simulink model "controller_2014B"  (R2014b)
settings: Solver=ode45  StartTime=0.0  StopTime=sim_run  FixedStep=0.001  RelTol=1e-3
InitFcn:
  | zh = 0.01;
undefined symbols (not defined in the file): Standard_Devices, UDP_Protocol, zh_step
libraries: rtwinlib x6, simulink x4, dspnetwork x2
settings Model: Creator=Lenka  LastModifiedBy=petrhomolka
settings DebuggingCC: FrameProcessingCompatibilityMsg=error

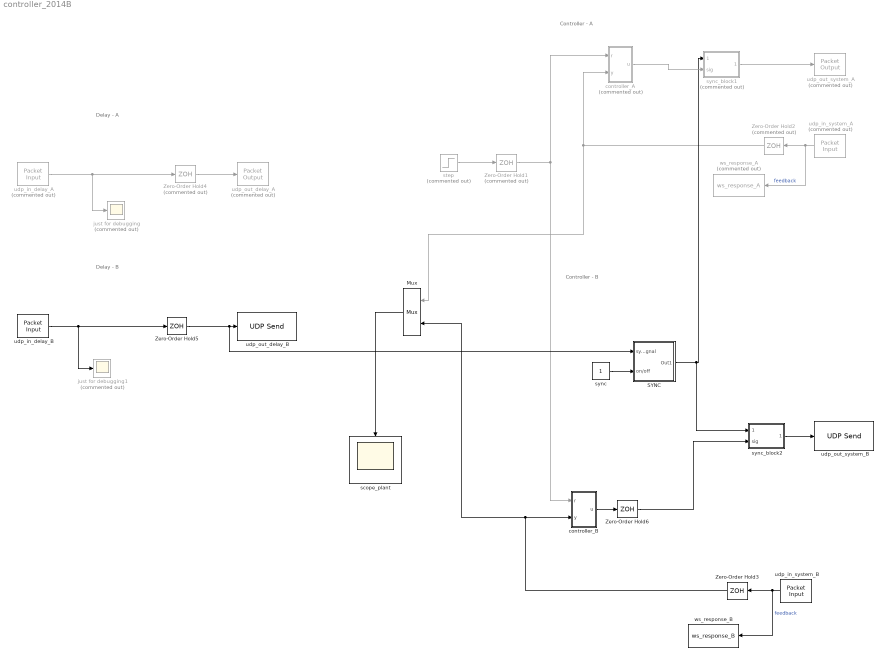
== system controller_2014B ==
  note: Controller - B
  note: Controller - A
  note: Delay - A
  note: Delay - B
  Mux : Mux  Inputs=2
  SYNC : Subsystem
  Zero-Order Hold1 : ZeroOrderHold  Commented=on  SampleTime=zh_step
  Zero-Order Hold2 : ZeroOrderHold  Commented=on  SampleTime=zh_step
  Zero-Order Hold3 : ZeroOrderHold  SampleTime=zh_step
  Zero-Order Hold4 : ZeroOrderHold  Commented=on  SampleTime=zh_step
  Zero-Order Hold5 : ZeroOrderHold  SampleTime=zh_step
  Zero-Order Hold6 : ZeroOrderHold  SampleTime=zh_step
  controller_A : Subsystem  Commented=on
  controller_B : Subsystem
  just for debugging : Scope  Commented=on
      settings: TimeRange=auto  LimitDataPoints=on  MaxDataPoints=5000  SaveToWorkspace=off  YMin=-10  YMax=10  SampleTime=-1  DataFormat=Array
  just for debugging1 : Scope  Commented=on
      settings: TimeRange=auto  LimitDataPoints=on  MaxDataPoints=5000  SaveToWorkspace=off  SaveName=ScopeData2  YMin=-10  YMax=10  SampleTime=-1  DataFormat=Array
  scope_plant : Scope
      settings: TimeRange=auto  ShowLegends=on  MaxDataPoints=5000  SaveToWorkspace=off  YMin=-63.375  YMax=570.375  SampleTime=-1
  step : Step  Commented=on  After=0.15  SampleTime=0
  sync : Constant
  sync_block1 : Subsystem  Commented=on
  sync_block2 : Subsystem
  udp_in_delay_A : rtwinlib/Packet Input  Commented=on  SampleTime=0.001  MaxMissedTicks=inf  ShowMissedTicks=off  YieldWhenWaiting=off  DrvName=Standard_Devices/UDP_Protocol  DrvAddress=28000  DrvOptions=[2468394752 28000]  PacketSize=8  DataTypes='double'  ShowReady=off  ShowError=off  PacketID=1  ByteOrder=1  ShowTimestamp=off
      settings: AttributesFormatString=Standard Devices\nUDP Protocol [6978h]
  udp_in_delay_B : rtwinlib/Packet Input  SampleTime=0.001  MaxMissedTicks=inf  ShowMissedTicks=off  YieldWhenWaiting=off  DrvName=Standard_Devices/UDP_Protocol  DrvAddress=28010  DrvOptions=[2164949811 28010]  PacketSize=8  DataTypes='double'  ShowReady=off  ShowError=off  PacketID=1  ByteOrder=1  ShowTimestamp=off
      settings: AttributesFormatString=Standard Devices\nUDP Protocol [6982h]
  udp_in_system_A : rtwinlib/Packet Input  Commented=on  SampleTime=0.001  MaxMissedTicks=inf  ShowMissedTicks=off  YieldWhenWaiting=off  DrvName=Standard_Devices/UDP_Protocol  DrvAddress=28500  DrvOptions=[2468394752 28500]  PacketSize=8  DataTypes='double'  ShowReady=off  ShowError=off  PacketID=1  ByteOrder=1  ShowTimestamp=off
      settings: AttributesFormatString=Standard Devices\nUDP Protocol [6F54h]
  udp_in_system_B : rtwinlib/Packet Input  SampleTime=0.001  MaxMissedTicks=inf  ShowMissedTicks=off  YieldWhenWaiting=off  DrvName=Standard_Devices/UDP_Protocol  DrvAddress=28510  DrvOptions=[2164949811 28510]  PacketSize=8  DataTypes='double'  ShowReady=off  ShowError=off  PacketID=1  ByteOrder=1  ShowTimestamp=off
      settings: AttributesFormatString=Standard Devices\nUDP Protocol [6F54h]
  udp_out_delay_A : rtwinlib/Packet Output  Commented=on  SampleTime=0.01  MaxMissedTicks=inf  ShowMissedTicks=off  YieldWhenWaiting=off  DrvName=Standard_Devices/UDP_Protocol  DrvAddress=27000  DrvOptions=[2468394752 27000]  PacketSize=8  DataTypes='double'  ShowReady=off  ShowError=off  PacketID=1  ByteOrder=1  InitialValue=[]  FinalValue=[]
      settings: AttributesFormatString=Standard Devices\nUDP Protocol [6D60h]
  udp_out_delay_B : dspnetwork/UDP Send  remoteURL='129.10.131.51'  remotePort=27010  localURL='0.0.0.0'  localPortSource=Automatically determine  localPort=27000  sampletime=-1  separateLengthPort=0
  udp_out_system_A : rtwinlib/Packet Output  Commented=on  SampleTime=0.01  MaxMissedTicks=inf  ShowMissedTicks=off  YieldWhenWaiting=off  DrvName=Standard_Devices/UDP_Protocol  DrvAddress=27500  DrvOptions=[2468394752 27500]  PacketSize=8  DataTypes='double'  ShowReady=off  ShowError=off  PacketID=1  ByteOrder=1  InitialValue=[]  FinalValue=[]
      settings: AttributesFormatString=Standard Devices\nUDP Protocol [6B6Ch]
  udp_out_system_B : dspnetwork/UDP Send  remoteURL='129.10.131.51'  remotePort=27510  localURL='0.0.0.0'  localPortSource=Automatically determine  localPort=27000  sampletime=-1  separateLengthPort=0
  ws_response_A : ToWorkspace  Commented=on  VariableName=ws_response_A  SaveFormat=Timeseries  SampleTime=zh_step
  ws_response_B : ToWorkspace  VariableName=ws_response_B  SaveFormat=Timeseries  SampleTime=zh_step
  wires:
  udp_in_system_A/1 -> ws_response_A/1, Zero-Order Hold2/1  "feedback"
  step/1 -> Zero-Order Hold1/1
  udp_in_system_B/1 -> ws_response_B/1, Zero-Order Hold3/1  "feedback"
  Mux/1 -> scope_plant/1
  Zero-Order Hold1/1 -> controller_A/1(r), controller_B/1(r)
  Zero-Order Hold2/1 -> controller_A/2(y), Mux/1
  udp_in_delay_A/1 -> just for debugging/1, Zero-Order Hold4/1
  Zero-Order Hold4/1 -> udp_out_delay_A/1
  udp_in_delay_B/1 -> just for debugging1/1, Zero-Order Hold5/1
  controller_B/1(u) -> Zero-Order Hold6/1
  sync_block2/1(sig out) -> udp_out_system_B/1
  Zero-Order Hold3/1 -> controller_B/2(y), Mux/2
  Zero-Order Hold5/1 -> SYNC/1(sync signal), udp_out_delay_B/1
  SYNC/1(Out1) -> sync_block2/1(sync_sig), sync_block1/1(sync_sig)
  sync_block1/1(sig out) -> udp_out_system_A/1
  controller_A/1(u) -> sync_block1/2(sig)
  sync/1 -> SYNC/2(on/off)
  Zero-Order Hold6/1 -> sync_block2/2(sig)

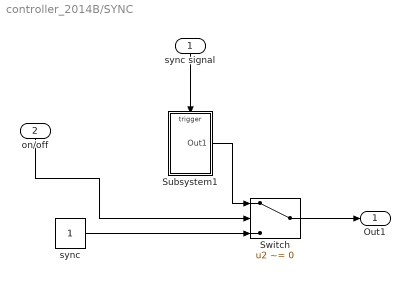
== system controller_2014B/SYNC ==
  sync signal : Inport
  on/off : Inport  Port=2
  Subsystem1 : Subsystem
  Switch : Switch  Criteria=u2 ~= 0
  sync : Constant
  Out1 : Outport
  wires:
  sync/1 -> Switch/3
  sync signal/1 -> Subsystem1/Trigger
  Subsystem1/1(Out1) -> Switch/1
  Switch/1 -> Out1/1
  on/off/1 -> Switch/2

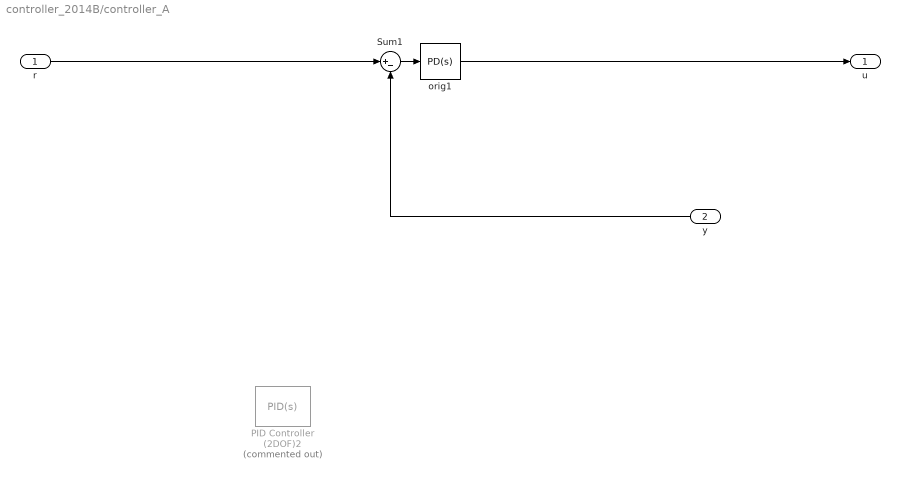
== system controller_2014B/controller_A ==
  r : Inport
  y : Inport  Port=2
  PID Controller (2DOF)2 : simulink/Continuous/PID Controller (2DOF)  Commented=on  Controller=PID  TimeDomain=Continuous-time  SampleTime=-1  IntegratorMethod=Forward Euler  FilterMethod=Forward Euler  Form=Parallel  UseFilter=on  ControllerParametersSource=internal  P=6.3799380872686  I=2.12979603411331  D=3.6093223618413  N=48.5068620404972  b=2.39624043732871  c=0.716079145801974  InitialConditionSource=internal  InitialConditionForIntegrator=0  InitialConditionForFilter=0  ExternalReset=none  LimitOutput=off  UpperSaturationLimit=inf  LowerSaturationLimit=-inf  LinearizeAsGain=on  AntiWindupMode=none  Kb=1  TrackingMode=off  Kt=1  PParamMin=[]  PParamMax=[]  IParamMin=[]  IParamMax=[]  DParamMin=[]  DParamMax=[]  NParamMin=[]  NParamMax=[]  bParamMin=[]  bParamMax=[]  cParamMin=[]  cParamMax=[]  KbParamMin=[]  KbParamMax=[]  KtParamMin=[]  KtParamMax=[]  POutMin=[]  POutMax=[]  IOutMin=[]  IOutMax=[]  DOutMin=[]  DOutMax=[]  NOutMin=[]  NOutMax=[]  bOutMin=[]  bOutMax=[]  cOutMin=[]  cOutMax=[]  KbOutMin=[]  KbOutMax=[]  KtOutMin=[]  KtOutMax=[]  IntegratorOutMin=[]  IntegratorOutMax=[]  FilterOutMin=[]  FilterOutMax=[]  SumOutMin=[]  SumOutMax=[]  Sum1OutMin=[]  Sum1OutMax=[]  Sum2OutMin=[]  Sum2OutMax=[]  Sum3OutMin=[]  Sum3OutMax=[]  SumI1OutMin=[]  SumI1OutMax=[]  SumI2OutMin=[]  SumI2OutMax=[]  SumI3OutMin=[]  SumI3OutMax=[]  SumDOutMin=[]  SumDOutMax=[]  SaturationOutMin=[]  SaturationOutMax=[]  IntegratorContinuousStateAttributes=''  IntegratorStateMustResolveToSignalObject=off  IntegratorRTWStateStorageClass=Auto  FilterContinuousStateAttributes=''  FilterStateMustResolveToSignalObject=off  FilterRTWStateStorageClass=Auto  DifferentiatorICPrevScaledInput=0  DifferentiatorOutMin=[]  DifferentiatorOutMax=[]
  Sum1 : Sum  Inputs=|+-
  orig1 : simulink/Continuous/PID Controller  Controller=PD  TimeDomain=Continuous-time  SampleTime=-1  IntegratorMethod=Forward Euler  FilterMethod=Forward Euler  Form=Parallel  UseFilter=on  ControllerParametersSource=internal  P=0.0142  I=0.0175856984919557  D=0.0001  N=100  InitialConditionSource=internal  InitialConditionForIntegrator=0  InitialConditionForFilter=0  ExternalReset=none  LimitOutput=on  UpperSaturationLimit=5/1000  LowerSaturationLimit=-5/1000  LinearizeAsGain=on  AntiWindupMode=none  Kb=1  TrackingMode=off  Kt=1  PParamMin=[]  PParamMax=[]  IParamMin=[]  IParamMax=[]  DParamMin=[]  DParamMax=[]  NParamMin=[]  NParamMax=[]  KbParamMin=[]  KbParamMax=[]  KtParamMin=[]  KtParamMax=[]  POutMin=[]  POutMax=[]  IOutMin=[]  IOutMax=[]  DOutMin=[]  DOutMax=[]  NOutMin=[]  NOutMax=[]  KbOutMin=[]  KbOutMax=[]  KtOutMin=[]  KtOutMax=[]  IntegratorOutMin=[]  IntegratorOutMax=[]  FilterOutMin=[]  FilterOutMax=[]  SumOutMin=[]  SumOutMax=[]  SumI1OutMin=[]  SumI1OutMax=[]  SumI2OutMin=[]  SumI2OutMax=[]  SumI3OutMin=[]  SumI3OutMax=[]  SumDOutMin=[]  SumDOutMax=[]  SaturationOutMin=[]  SaturationOutMax=[]  IntegratorContinuousStateAttributes=''  IntegratorStateMustResolveToSignalObject=off  IntegratorRTWStateStorageClass=Auto  FilterContinuousStateAttributes=''  FilterStateMustResolveToSignalObject=off  FilterRTWStateStorageClass=Auto  DifferentiatorICPrevScaledInput=0  DifferentiatorOutMin=[]  DifferentiatorOutMax=[]
  u : Outport
  wires:
  orig1/1 -> u/1
  y/1 -> Sum1/2
  r/1 -> Sum1/1
  Sum1/1 -> orig1/1

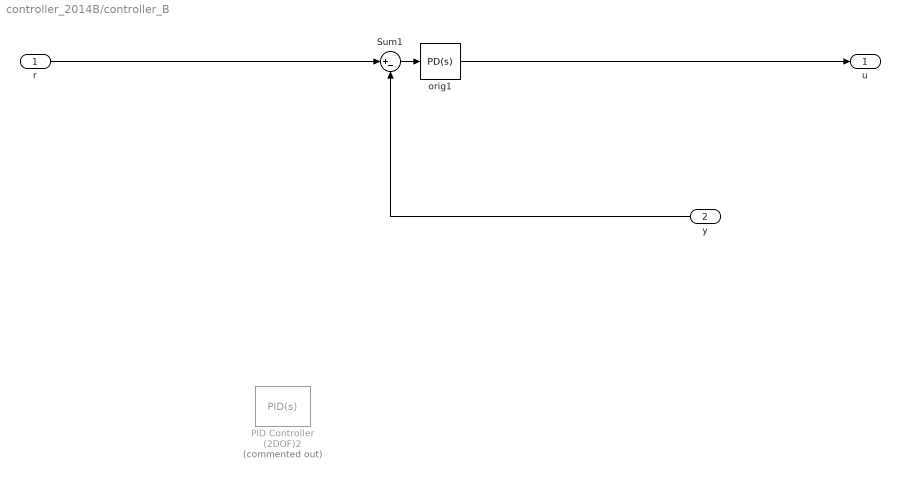
== system controller_2014B/controller_B ==
  r : Inport
  y : Inport  Port=2
  PID Controller (2DOF)2 : simulink/Continuous/PID Controller (2DOF)  Commented=on  Controller=PID  TimeDomain=Continuous-time  SampleTime=-1  IntegratorMethod=Forward Euler  FilterMethod=Forward Euler  Form=Parallel  UseFilter=on  ControllerParametersSource=internal  P=6.3799380872686  I=2.12979603411331  D=3.6093223618413  N=48.5068620404972  b=2.39624043732871  c=0.716079145801974  InitialConditionSource=internal  InitialConditionForIntegrator=0  InitialConditionForFilter=0  ExternalReset=none  LimitOutput=off  UpperSaturationLimit=inf  LowerSaturationLimit=-inf  LinearizeAsGain=on  AntiWindupMode=none  Kb=1  TrackingMode=off  Kt=1  PParamMin=[]  PParamMax=[]  IParamMin=[]  IParamMax=[]  DParamMin=[]  DParamMax=[]  NParamMin=[]  NParamMax=[]  bParamMin=[]  bParamMax=[]  cParamMin=[]  cParamMax=[]  KbParamMin=[]  KbParamMax=[]  KtParamMin=[]  KtParamMax=[]  POutMin=[]  POutMax=[]  IOutMin=[]  IOutMax=[]  DOutMin=[]  DOutMax=[]  NOutMin=[]  NOutMax=[]  bOutMin=[]  bOutMax=[]  cOutMin=[]  cOutMax=[]  KbOutMin=[]  KbOutMax=[]  KtOutMin=[]  KtOutMax=[]  IntegratorOutMin=[]  IntegratorOutMax=[]  FilterOutMin=[]  FilterOutMax=[]  SumOutMin=[]  SumOutMax=[]  Sum1OutMin=[]  Sum1OutMax=[]  Sum2OutMin=[]  Sum2OutMax=[]  Sum3OutMin=[]  Sum3OutMax=[]  SumI1OutMin=[]  SumI1OutMax=[]  SumI2OutMin=[]  SumI2OutMax=[]  SumI3OutMin=[]  SumI3OutMax=[]  SumDOutMin=[]  SumDOutMax=[]  SaturationOutMin=[]  SaturationOutMax=[]  IntegratorContinuousStateAttributes=''  IntegratorStateMustResolveToSignalObject=off  IntegratorRTWStateStorageClass=Auto  FilterContinuousStateAttributes=''  FilterStateMustResolveToSignalObject=off  FilterRTWStateStorageClass=Auto  DifferentiatorICPrevScaledInput=0  DifferentiatorOutMin=[]  DifferentiatorOutMax=[]
  Sum1 : Sum  Inputs=|+-
  orig1 : simulink/Continuous/PID Controller  Controller=PD  TimeDomain=Continuous-time  SampleTime=-1  IntegratorMethod=Forward Euler  FilterMethod=Forward Euler  Form=Parallel  UseFilter=on  ControllerParametersSource=internal  P=0.0142  I=0.0175856984919557  D=0.0001  N=100  InitialConditionSource=internal  InitialConditionForIntegrator=0  InitialConditionForFilter=0  ExternalReset=none  LimitOutput=on  UpperSaturationLimit=5/1000  LowerSaturationLimit=-5/1000  LinearizeAsGain=on  AntiWindupMode=none  Kb=1  TrackingMode=off  Kt=1  PParamMin=[]  PParamMax=[]  IParamMin=[]  IParamMax=[]  DParamMin=[]  DParamMax=[]  NParamMin=[]  NParamMax=[]  KbParamMin=[]  KbParamMax=[]  KtParamMin=[]  KtParamMax=[]  POutMin=[]  POutMax=[]  IOutMin=[]  IOutMax=[]  DOutMin=[]  DOutMax=[]  NOutMin=[]  NOutMax=[]  KbOutMin=[]  KbOutMax=[]  KtOutMin=[]  KtOutMax=[]  IntegratorOutMin=[]  IntegratorOutMax=[]  FilterOutMin=[]  FilterOutMax=[]  SumOutMin=[]  SumOutMax=[]  SumI1OutMin=[]  SumI1OutMax=[]  SumI2OutMin=[]  SumI2OutMax=[]  SumI3OutMin=[]  SumI3OutMax=[]  SumDOutMin=[]  SumDOutMax=[]  SaturationOutMin=[]  SaturationOutMax=[]  IntegratorContinuousStateAttributes=''  IntegratorStateMustResolveToSignalObject=off  IntegratorRTWStateStorageClass=Auto  FilterContinuousStateAttributes=''  FilterStateMustResolveToSignalObject=off  FilterRTWStateStorageClass=Auto  DifferentiatorICPrevScaledInput=0  DifferentiatorOutMin=[]  DifferentiatorOutMax=[]
  u : Outport
  wires:
  orig1/1 -> u/1
  y/1 -> Sum1/2
  r/1 -> Sum1/1
  Sum1/1 -> orig1/1

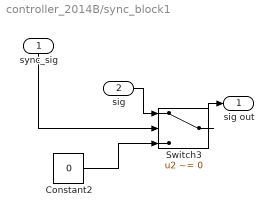
== system controller_2014B/sync_block1 ==
  sync_sig : Inport
  sig : Inport  Port=2
  Constant2 : Constant  Value=0
  Switch3 : Switch  Criteria=u2 ~= 0
  sig out : Outport
  wires:
  sync_sig/1 -> Switch3/2
  Switch3/1 -> sig out/1
  sig/1 -> Switch3/1
  Constant2/1 -> Switch3/3

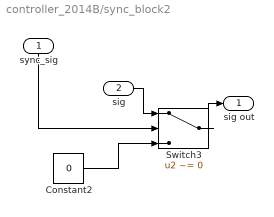
== system controller_2014B/sync_block2 ==
  sync_sig : Inport
  sig : Inport  Port=2
  Constant2 : Constant  Value=0
  Switch3 : Switch  Criteria=u2 ~= 0
  sig out : Outport
  wires:
  Constant2/1 -> Switch3/3
  sig/1 -> Switch3/1
  Switch3/1 -> sig out/1
  sync_sig/1 -> Switch3/2

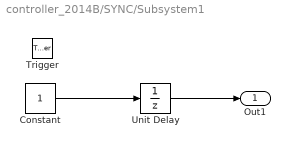
== system controller_2014B/SYNC/Subsystem1 ==
  Trigger : TriggerPort  PortDimensions=1
  Constant : Constant
  Unit Delay : UnitDelay  SampleTime=-1
  Out1 : Outport
  wires:
  Unit Delay/1 -> Out1/1
  Constant/1 -> Unit Delay/1
